simulink model "CollectorUnglazedISO9806_2node"  (R2018b)
settings: Solver=ode45  StartTime=0.0  StopTime=4*24*3600  RelTol=1e-5  AbsTol=1e-5  EnableMultiTasking=on
undefined symbols (not defined in the file): path_carnot
libraries: carnot x8, simulink x2
settings Model: Creator=drhf  LastModifiedBy=drhf
settings SolverCC: AutoScaleAbsTol=off
settings DataIOCC: LimitDataPoints=on  SaveFormat=Array
settings OptimizationCC: ExpressionDepthLimit=2147483647  LifeSpan=inf
settings DebuggingCC: UnderspecifiedInitializationDetection=Classic  MergeDetectMultiDrivingBlocksExec=none  SolverPrmCheckMsg=warning  StateNameClashWarn=warning  SFUnexpectedBacktrackingDiag=warning  SFNoUnconditionalDefaultTransitionDiag=warning  SFExecutionAtInitializationDiag=none
settings HardwareCC: ProdBitPerPointer=32  ProdBitPerSizeT=32  ProdBitPerPtrDiffT=32  ProdLargestAtomicFloat=None  ProdIntDivRoundTo=Undefined  ProdEndianess=Unspecified  ProdWordSize=32  ProdHWDeviceType=32-bit Generic
settings ModelReferenceCC: PropagateSignalLabelsOutOfModel=off
settings SFSimCC: SimUseLocalCustomCode=off
settings RTWCC: RTWUseLocalCustomCode=off
settings CodeAppCC: StateflowObjectComments=on
settings GRTTargetCC: TargetLangStandard=C89/C90 (ANSI)  GeneratePreprocessorConditionals=Disable all  CombineOutputUpdateFcns=off  GRTInterface=on
settings ConfigComp: CovMetricSettings=dw  CovHtmlReporting=on  CovSaveCumulativeToWorkspaceVar=on  CovSaveSingleToWorkspaceVar=on  CovExternalEMLEnable=off

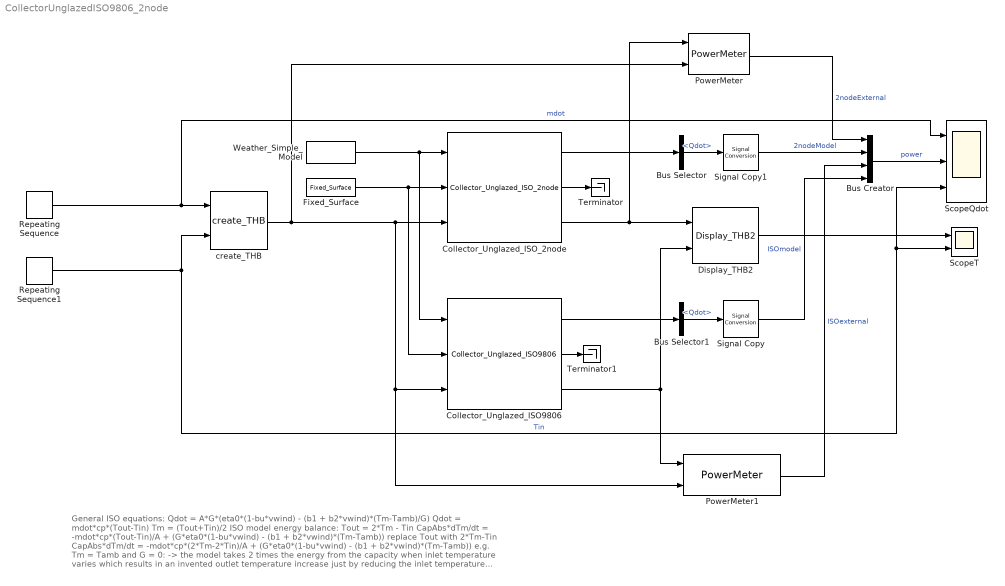
== system CollectorUnglazedISO9806_2node ==
  note: General ISO equations:
      | Qdot = A*G*(eta0*(1-bu*vwind) - (b1 + b2*vwind)*(Tm-Tamb)/G)
      | Qdot = mdot*cp*(Tout-Tin)
      | Tm = (Tout+Tin)/2
      |
      | ISO model energy balance:
      | Tout = 2*Tm - Tin
      | CapAbs*dTm/dt = -mdot*cp*(Tout-Tin)/A + (G*eta0*(1-bu*vwind) - (b1 + b2*vwind)*(Tm-Tamb))
      | replace Tout with 2*Tm-Tin
      | CapAbs*dTm/dt = -mdot*cp*(2*Tm-2*Tin)/A + (G*eta0*(1-bu*vwind) - (b1 + b2*vwind)*(Tm-Tamb))
      | e.g. Tm = Tamb and G = 0:
      | -> the model takes 2 times the energy from the capacity when inlet temperature varies
      | which results in an invented outlet temperature increase just by reducing the inlet temperature
      |
      | Modified 2 node model energy balance:
      | Acol*Ncol*CapAbs/2 * dTin/dt = mdot*cp*(Tinlet-Tin)
      | CapAbs/2 * dTout/dt = -mdot*cp*(Tout-Tin)/(Acol*Ncol) + (G*eta0*(1-bu*vwind) - (b1 + b2*vwind)*(Tm-Tamb))
  Bus Creator : BusCreator  Inputs=4
  Bus Selector : BusSelector  OutputSignals=Qdot
  Bus Selector1 : BusSelector  OutputSignals=Qdot
  Collector_Unglazed_ISO9806 : carnot/Source/Solar_Thermal/Collector_Unglazed_ISO9806  tini=20  Ncollector=2  PathName=fullfile(path_carnot('libsl'), 'Source', 'Solar_Thermal', 'Collector_Unglazed_ISO9806', 'parameter_set')  FileName='Viessmann_SLK_ISO9806.mat'  userPath=off  userParam=off  acol=2.544  len=2.1  eta0=0.702  bu=0.066  b1=32.64  b2=3.59  c_abs=50*3900  dplin=5504.4  dpqua=6222.096
      settings: SourceProductName=Carnot
  Collector_Unglazed_ISO_2node : carnot/Source/Solar_Thermal/Collector_Unglazed_ISO_2node  tini=20  Ncollector=2  PathName=fullfile(path_carnot('libsl'), 'Source', 'Solar_Thermal', 'Collector_Unglazed_ISO9806', 'parameter_set')  FileName='Viessmann_SLK_ISO9806.mat'  userPath=off  userParam=off  acol=2.544  len=2.1  eta0=0.702  bu=0.066  b1=32.64  b2=3.59  c_abs=50*3900  dplin=5504.4  dpqua=6222.096
      settings: SourceProductName=Carnot
  Display_THB2 : carnot/Outputs/Display_THB2  t=on  m=off  p=off  id=off  mix=off  d=off
      settings: SourceProductName=Carnot
  Fixed_Surface : carnot/Weather/Fixed_Surface  colangle=30  colazi=0  colrot=0
      settings: SourceProductName=Carnot
  PowerMeter : carnot/Control/PowerMeter
      settings: SourceProductName=Carnot
  PowerMeter1 : carnot/Control/PowerMeter
      settings: SourceProductName=Carnot
  Repeating Sequence : simulink/Sources/Repeating Sequence  rep_seq_t=[0 24 36 48 60 100]*3600  rep_seq_y=[126 126 10 126 126 126]/3600
  Repeating Sequence1 : simulink/Sources/Repeating Sequence  rep_seq_t=[0 24 36 48 60 100]*3600  rep_seq_y=[20 20 20 20 5 5]
  ScopeQdot : Scope  NumInputPorts=3
  ScopeT : Scope  NumInputPorts=2
  Signal Copy : SignalConversion  OverrideOpt=off
  Signal Copy1 : SignalConversion  OverrideOpt=off
  Terminator : Terminator
  Terminator1 : Terminator
  Weather_Simple_Model : carnot/Weather/Weather_Simple_Model  Ibn=900  Idg=100  tamb=20  deltaTsky=0  rh=50  precip="10e-3/24/3600           % 10 mm in 24 h"  cloud=0.125  p=1013e2  vw=1  wdir=270  lat=60  colangle=0  colazi=0  colrot=0
      settings: SourceProductName=Carnot
  create_THB : carnot/Source/Simple/create_THB  p=1e5  fluid=Water  mix=0  mix2=0  mix3=0  dia=0  hgt=0  mID=No Pressure Drop
      settings: SourceProductName=Carnot
  wires:
  Weather_Simple_Model/1 -> Collector_Unglazed_ISO_2node/1, Collector_Unglazed_ISO9806/1
  Fixed_Surface/1 -> Collector_Unglazed_ISO_2node/2, Collector_Unglazed_ISO9806/2
  create_THB/1 -> PowerMeter/2, Collector_Unglazed_ISO_2node/3, PowerMeter1/2, Collector_Unglazed_ISO9806/3
  Collector_Unglazed_ISO_2node/3 -> PowerMeter/1, Display_THB2/1
  Display_THB2/1 -> ScopeT/1
  Collector_Unglazed_ISO_2node/1 -> Bus Selector/1
  Collector_Unglazed_ISO_2node/2 -> Terminator/1
  Collector_Unglazed_ISO9806/1 -> Bus Selector1/1
  Collector_Unglazed_ISO9806/2 -> Terminator1/1
  Collector_Unglazed_ISO9806/3 -> PowerMeter1/1, Display_THB2/2
  Bus Selector/1 -> Signal Copy1/1  "<Qdot>"
  Bus Selector1/1 -> Signal Copy/1  "<Qdot>"
  Bus Creator/1 -> ScopeQdot/2  "power"
  Repeating Sequence1/1 -> ScopeQdot/3, ScopeT/2, create_THB/2  "Tin"
  Repeating Sequence/1 -> ScopeQdot/1, create_THB/1  "mdot"
  Signal Copy/1 -> Bus Creator/4  "ISOmodel"
  Signal Copy1/1 -> Bus Creator/2  "2nodeModel"
  PowerMeter/1 -> Bus Creator/1  "2nodeExternal"
  PowerMeter1/1 -> Bus Creator/3  "ISOexternal"
